simulink model "verify_Ventilation_Window_mdl"  (R2016b)
settings: Solver=VariableStepDiscrete  StartTime=0  StopTime=100  MaxStep=1  RelTol=1e-3  EnableMultiTasking=on
libraries: simulink x1, carnot x1
settings Model: Creator=drhf  LastModifiedBy=User
settings DataIOCC: SaveFormat=Array  SignalLoggingSaveFormat=ModelDataLogs
settings OptimizationCC: ExpressionDepthLimit=2147483647  LifeSpan=inf
settings DebuggingCC: UnderspecifiedInitializationDetection=Classic  MergeDetectMultiDrivingBlocksExec=none  SolverPrmCheckMsg=warning  FcnCallInpInsideContextMsg=warning  StateNameClashWarn=warning  SFUnexpectedBacktrackingDiag=warning  SFNoUnconditionalDefaultTransitionDiag=warning  SFExecutionAtInitializationDiag=none
settings HardwareCC: ProdBitPerPointer=32  ProdBitPerSizeT=32  ProdBitPerPtrDiffT=32  ProdLargestAtomicFloat=None  ProdIntDivRoundTo=Undefined  ProdEndianess=Unspecified  ProdWordSize=32  ProdHWDeviceType=32-bit Generic
settings ModelReferenceCC: PropagateSignalLabelsOutOfModel=off
settings GRTTargetCC: TargetLangStandard=C89/C90 (ANSI)  GeneratePreprocessorConditionals=Disable all  CombineOutputUpdateFcns=off  GRTInterface=on
settings ConfigComp: CovMetricSettings=dw  CovHtmlReporting=on  CovSaveCumulativeToWorkspaceVar=on  CovSaveSingleToWorkspaceVar=on  CovExternalEMLEnable=off

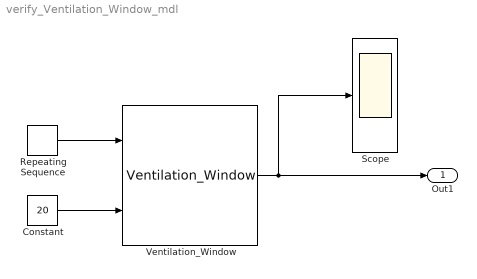
== system verify_Ventilation_Window_mdl ==
  Constant : Constant  Value=20
  Repeating Sequence : simulink/Sources/Repeating Sequence  rep_seq_t=[0 20 30 60 70 100]  rep_seq_y=[10 10 25 25 30 30]
  Scope : Scope
  Ventilation_Window : carnot/Source/Ventilation/Ventilation_Window  vent=0.4  rec=0.6  Vhouse=140*2.6
  Out1 : Outport
  wires:
  Ventilation_Window/1 -> Out1/1, Scope/1
  Constant/1 -> Ventilation_Window/2
  Repeating Sequence/1 -> Ventilation_Window/1
